simulink model "motor_sim"  (R2022b)
settings: Solver=VariableStepAuto  StartTime=0.0  StopTime=10.0  RelTol=1e-3
values from neighbouring files (symbols this model uses):
  B = Km*I/No_Load_rad    (= 6.49608448082e-07)    [motor_params.m]
  J = 9.06*10^-7    (= 9.06e-07)    [motor_params.m]
  Kb = 9.73*10^-3    (= 0.00973)    [motor_params.m]
  Km = 9.73*10^-3    (= 0.00973)    [motor_params.m]
  L = 0.035*10^-3    (= 3.5e-05)    [motor_params.m]
  R = 0.335    [motor_params.m]
settings Model: Creator=alice  LastModifiedBy=alice

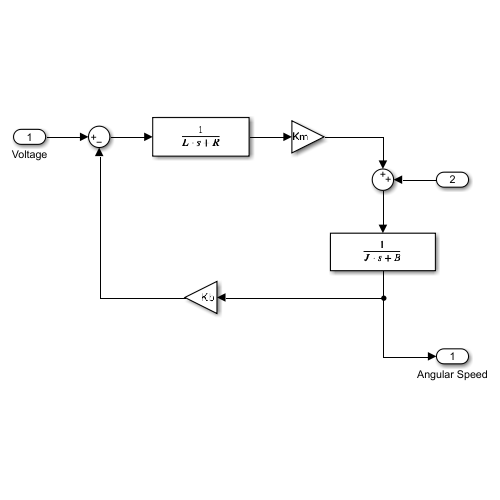
[thumbnail: Simulink's stored preview of the top-level diagram]
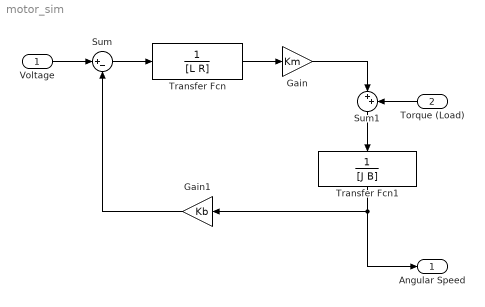
== system motor_sim ==
  Voltage : Inport
  Torque (Load) : Inport  Port=2
  Gain : Gain  Gain=Km
  Gain1 : Gain  Gain=Kb
  Sum : Sum  Inputs=|+-
  Sum1 : Sum  Inputs=|++
  Transfer Fcn : TransferFcn  Denominator=[L R]
  Transfer Fcn1 : TransferFcn  Denominator=[J B]
  Angular Speed : Outport
  wires:
  Voltage/1 -> Sum/1
  Sum/1 -> Transfer Fcn/1
  Transfer Fcn/1 -> Gain/1
  Transfer Fcn1/1 -> Gain1/1, Angular Speed/1
  Sum1/1 -> Transfer Fcn1/1
  Gain/1 -> Sum1/1
  Torque (Load)/1 -> Sum1/2
  Gain1/1 -> Sum/2
